simulink model "Dynamic_obstacle_avoidance"  (R2019a)
settings: Solver=VariableStepAuto  StartTime=0.0  StopTime=distance/V  MaxStep=1e-3  RelTol=1e-3  EnableMultiTasking=on
undefined symbols (not defined in the file): extended_map, Lw, obstacle, p, param, Ts, u0, WMV, WMVR, WOV, x0_dyn
libraries: simulink x2, mpclib x1
settings Model: Creator=The MathWorks, Inc.  LastModifiedBy=djtn
settings SolverCC: AlgebraicLoopSolver=LineSearch  MinimalZcImpactIntegration=on
settings DataIOCC: LimitDataPoints=on  SaveFormat=Array  SaveOutput=off  DSMLogging=off  SaveTime=off  ReturnWorkspaceOutputs=off
settings OptimizationCC: LifeSpan=inf
settings DebuggingCC: AlgebraicLoopMsg=none  UnderspecifiedInitializationDetection=Classic  MergeDetectMultiDrivingBlocksExec=none  SolverPrmCheckMsg=warning  AllowSymbolicDim=off  StateNameClashWarn=warning  SFUnexpectedBacktrackingDiag=warning  SFNoUnconditionalDefaultTransitionDiag=warning  SFExecutionAtInitializationDiag=none  UnderSpecifiedDimensionMsg=warning  ArithmeticOperatorsInVariantConditions=warning
settings HardwareCC: ProdBitPerPointer=32  ProdBitPerSizeT=32  ProdBitPerPtrDiffT=32  ProdLargestAtomicFloat=None  ProdIntDivRoundTo=Undefined  ProdEndianess=Unspecified  ProdWordSize=32  ProdHWDeviceType=32-bit Generic
settings ModelReferenceCC: PropagateSignalLabelsOutOfModel=off
settings SFSimCC: SimUseLocalCustomCode=off
settings RTWCC: RTWUseLocalCustomCode=off
settings CodeAppCC: StateflowObjectComments=on
settings GRTTargetCC: TargetLangStandard=C89/C90 (ANSI)
settings ConfigComp: CovMetricSettings=dw  CovSaveCumulativeToWorkspaceVar=on  CovSaveSingleToWorkspaceVar=on  CovExternalEMLEnable=off  CovSFcnEnable=off
settings SimscapeCC: SimscapeNormalizeSystem=off  SimscapeNominalValues="[{\"value\":\"10\",\"unit\":\"V\"},{\"value\":\"1\",\"unit\":\"A\"},{\"value\":\"10\",\"unit\":\"N*m\"},{\"value\":\"10\",\"unit\":\"bar\"},{\"value\":\"100\",\"unit\":\"kJ/kg\"},{\"value\":\"1\",\"unit\":\"kW\"},{\"value\":\"300\",\"unit\":\"K\"},{\"value\":\"100\",\"unit\":\"cm^3/s\"},{\"value\":\"1\",\"unit\":\"kN\"},{\"value\":\"1\",\"unit\":\"g/cm^3\"},{\"value\":\"1\",\"unit\":\"l\"},{\"value\":\"1\",\"unit\":\"cm^2\"},{\"value\":\"60\",\"unit\":\"Hz\"}]"
settings ConfigurationSet: Description=SimMechanics 2G
settings ExplorerConfigSet: InternalSimMechanicsExplorerSettings="<ExplorerConfiguration><canonicalview>default</canonicalview><AnimationSetting><BasePlaybackSpeed>1.0</BasePlaybackSpeed><PlaybackSpeedFactor>1.0</PlaybackSpeedFactor></AnimationSetting><TilePanel><TileInfo><Tiles Columns=\"1\" Count=\"1\" Rows=\"1\"><Column Left=\"2\" Weight=\"1\"/><Column Left=\"1552\"/><Row Top=\"2\" Weight=\"1\"/><Row Top=\"932\"/><Tile Height=\"1\" Width=\"1\" X=\"0\" Y=\"0\"/></Tiles></TileInfo><SceneInfo><SceneViewer><BGColor><R>0.60000002384185791</R><G>0.60000002384185791</G><B>0.60000002384185791</B></BGColor><Camera><Position><X>0.027865189060748197</X><Y>-2.5719092456962986</Y><Z>0.23157896538506753</Z></Position><Center><X>0.62659712312732463</X><Y>-0.46110119691712204</Y><Z>0.22087365386473376</Z></Center><Up><X>-0.0079438354874226333</X><Y>0.0073246425924307582</Y><Z>0.99994162084025784</Z></Up><Left>-0.24533778208815546</Left><Right>0.24533778208815546</Right><Bottom>-0.79734779727023208</Bottom><Top>0.79734779727023208</Top></Camera></SceneViewer></SceneInfo></TilePanel></ExplorerConfiguration>"

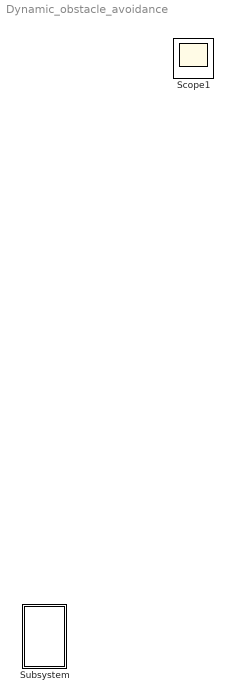
== system Dynamic_obstacle_avoidance ==
  Subsystem : Subsystem
  Scope1 : Scope

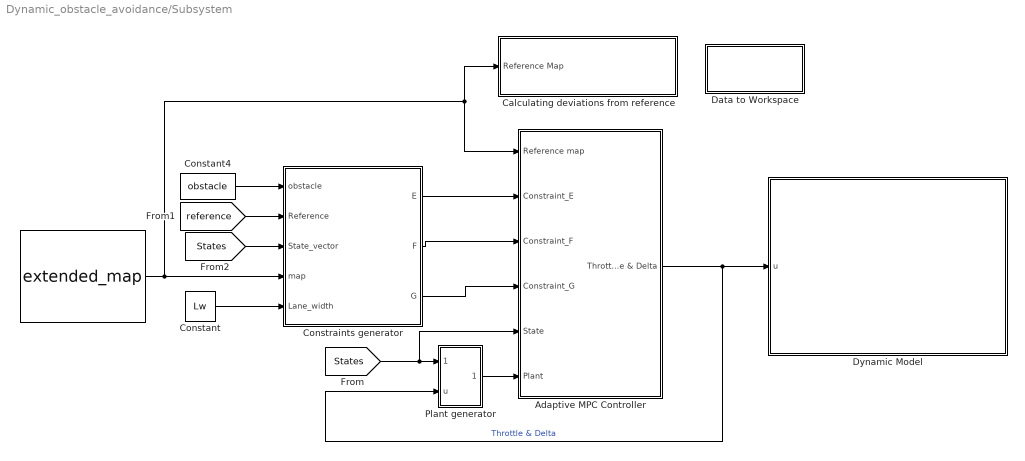
== system Dynamic_obstacle_avoidance/Subsystem ==
  "  " : Constant  Value=extended_map  SampleTime=Ts
      mask Display: image('creative_map_city.jpg')
  Adaptive MPC Controller : Subsystem
  Calculating deviations from reference : Subsystem
  Constant : Constant  Value=Lw
  Constant4 : Constant  Value=obstacle
  Constraints generator : Subsystem
  Data to Workspace : Subsystem
  Dynamic Model : Subsystem
      mask Display: image('hyundai_verna.jpg')
  Plant generator : Subsystem
  wires:
  Plant generator/1(Out1) -> Adaptive MPC Controller/6(Plant)
  Constraints generator/3(G) -> Adaptive MPC Controller/4(Constraint_G)
  "  "/1 -> Adaptive MPC Controller/1(Reference map), Calculating deviations from reference/1(Reference Map), Constraints generator/4(map)
  Adaptive MPC Controller/1(Throttle & Delta) -> Dynamic Model/1(u), Plant generator/2(u)  "Throttle & Delta"
  Constraints generator/1(E) -> Adaptive MPC Controller/2(Constraint_E)
  Constraints generator/2(F) -> Adaptive MPC Controller/3(Constraint_F)
  [States] -> Adaptive MPC Controller/5(State), Plant generator/1(State)
  Constant4/1 -> Constraints generator/1(obstacle)
  [reference] -> Constraints generator/2(Reference)
  Constant/1 -> Constraints generator/5(Lane_width)
  [States] -> Constraints generator/3(State_vector)

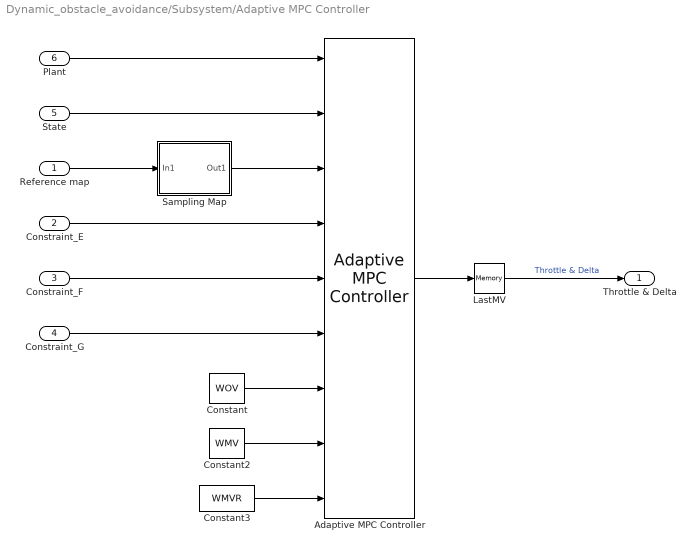
== system Dynamic_obstacle_avoidance/Subsystem/Adaptive MPC Controller ==
  Reference map : Inport
  Constraint_E : Inport  Port=2
  Constraint_F : Inport  Port=3
  Constraint_G : Inport  Port=4
  State : Inport  Port=5
  Plant : Inport  Port=6
  Adaptive MPC Controller : mpclib/Adaptive MPC Controller  SCDEnableBlockLinearizationSpecification=on  mpcobj=mpcobj  x0=egoStates  enable_value=0  updateMPCinCallerWorkspace=on  md_inport=off  mv_inport=off  uref_inport=off  return_cost=off  return_mvseq=off  return_qpstatus=off  return_xseq=off  return_state=off  return_ovseq=off  state_inport=off  isltv_plant=off  umin_inport=off  umax_inport=off  ymin_inport=off  ymax_inport=off  cc_inport=on  ywt_inport=on  uwt_inport=on  duwt_inport=on  rhoeps_inport=off  pm_inport=off  MaximumP=10  HorizonChoice=FixedHorizon  BlockDataType=double  SampleTimeInherited=on  switch_inport=off
  Constant : Constant  Value=WOV
  Constant2 : Constant  Value=WMV
  Constant3 : Constant  Value=WMVR
  LastMV : Memory  InitialCondition=u0
  Sampling Map : Subsystem
  Throttle & Delta : Outport  VectorParamsAs1DForOutWhenUnconnected=on
  wires:
  Constraint_E/1 -> Adaptive MPC Controller/4
  Constraint_G/1 -> Adaptive MPC Controller/6
  Constant3/1 -> Adaptive MPC Controller/9
  Constant2/1 -> Adaptive MPC Controller/8
  Constraint_F/1 -> Adaptive MPC Controller/5
  Constant/1 -> Adaptive MPC Controller/7
  State/1 -> Adaptive MPC Controller/2
  Adaptive MPC Controller/1 -> LastMV/1
  LastMV/1 -> Throttle & Delta/1  "Throttle & Delta"
  Plant/1 -> Adaptive MPC Controller/1
  Reference map/1 -> Sampling Map/1(In1)
  Sampling Map/1(Out1) -> Adaptive MPC Controller/3

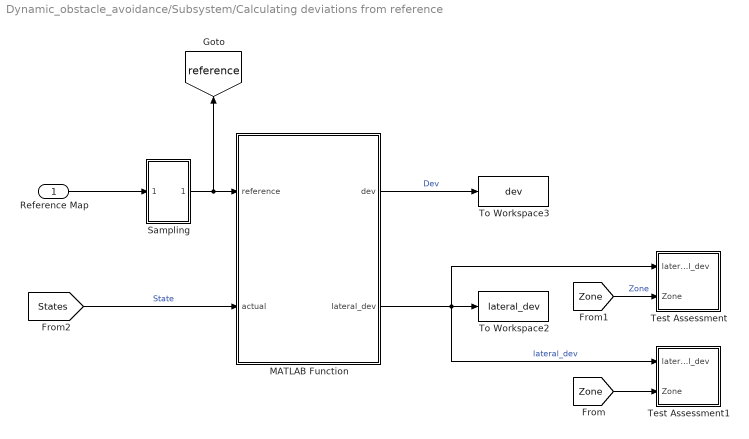
== system Dynamic_obstacle_avoidance/Subsystem/Calculating deviations from reference ==
  Reference Map : Inport
  MATLAB Function : MATLAB Function  TreatAsAtomicUnit=on
  Sampling : Subsystem
  Test Assessment : Test Sequence  TreatAsAtomicUnit=on
  Test Assessment1 : Test Sequence  TreatAsAtomicUnit=on
  To Workspace2 : ToWorkspace  VariableName=lateral_dev  SampleTime=Ts
  To Workspace3 : ToWorkspace  VariableName=dev  SampleTime=-1
  tag scope: reference=global
  wires:
  [Zone] -> Test Assessment1/2(Zone)
  [Zone] -> Test Assessment/2(Zone)  "Zone"
  MATLAB Function/2(lateral_dev) -> To Workspace2/1, Test Assessment/1(lateral_dev), Test Assessment1/1(lateral_dev)  "lateral_dev"
  MATLAB Function/1(dev) -> To Workspace3/1  "Dev"
  [States] -> MATLAB Function/2(actual)  "State"
  Reference Map/1 -> Sampling/1(In1)
  Sampling/1(Out1) -> MATLAB Function/1(reference), [reference]

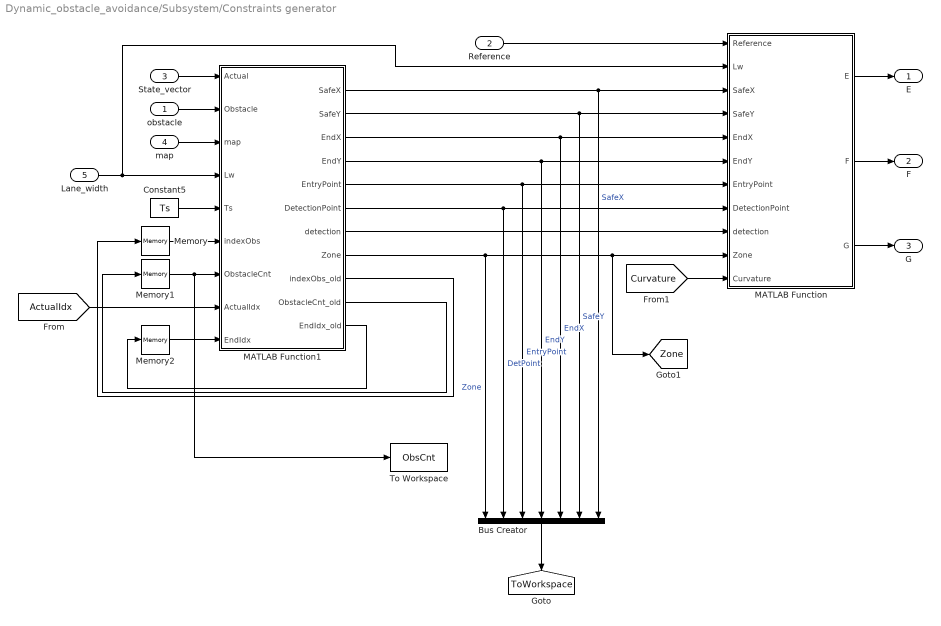
== system Dynamic_obstacle_avoidance/Subsystem/Constraints generator ==
  obstacle : Inport
  Reference : Inport  Port=2
  State_vector : Inport  Port=3
  map : Inport  Port=4
  Lane_width : Inport  Port=5
  Bus Creator : BusCreator  Inputs=7
  Constant5 : Constant  Value=Ts
  MATLAB Function : MATLAB Function  TreatAsAtomicUnit=on
  MATLAB Function1 : MATLAB Function  TreatAsAtomicUnit=on
  Memory : Memory
  Memory1 : Memory
  Memory2 : Memory
  To Workspace : ToWorkspace  VariableName=ObsCnt  SampleTime=Ts
  E : Outport  VectorParamsAs1DForOutWhenUnconnected=on
  F : Outport  Port=2  VectorParamsAs1DForOutWhenUnconnected=on
  G : Outport  Port=3  VectorParamsAs1DForOutWhenUnconnected=on
  tag scope: ToWorkspace=global, Zone=global
  wires:
  obstacle/1 -> MATLAB Function1/2(Obstacle)
  State_vector/1 -> MATLAB Function1/1(Actual)
  map/1 -> MATLAB Function1/3(map)
  Constant5/1 -> MATLAB Function1/5(Ts)
  Lane_width/1 -> MATLAB Function1/4(Lw), MATLAB Function/2(Lw)
  Memory/1 -> MATLAB Function1/6(indexObs)
  MATLAB Function1/9(indexObs_old) -> Memory/1
  MATLAB Function1/1(SafeX) -> Bus Creator/7, MATLAB Function/3(SafeX)  "SafeX"
  MATLAB Function1/2(SafeY) -> Bus Creator/6, MATLAB Function/4(SafeY)  "SafeY"
  MATLAB Function1/3(EndX) -> Bus Creator/5, MATLAB Function/5(EndX)  "EndX"
  MATLAB Function1/4(EndY) -> Bus Creator/4, MATLAB Function/6(EndY)  "EndY"
  MATLAB Function1/5(EntryPoint) -> Bus Creator/3, MATLAB Function/7(EntryPoint)  "EntryPoint"
  MATLAB Function1/6(DetectionPoint) -> Bus Creator/2, MATLAB Function/8(DetectionPoint)  "DetPoint"
  MATLAB Function1/7(detection) -> MATLAB Function/9(detection)
  MATLAB Function1/8(Zone) -> Bus Creator/1, MATLAB Function/10(Zone), [Zone]  "Zone"
  Reference/1 -> MATLAB Function/1(Reference)
  MATLAB Function/1(E) -> E/1
  MATLAB Function/2(F) -> F/1
  MATLAB Function/3(G) -> G/1
  Memory1/1 -> To Workspace/1, MATLAB Function1/7(ObstacleCnt)
  MATLAB Function1/10(ObstacleCnt_old) -> Memory1/1
  [ActualIdx] -> MATLAB Function1/8(ActualIdx)
  Memory2/1 -> MATLAB Function1/9(EndIdx)
  MATLAB Function1/11(EndIdx_old) -> Memory2/1
  Bus Creator/1 -> [ToWorkspace]
  [Curvature] -> MATLAB Function/11(Curvature)

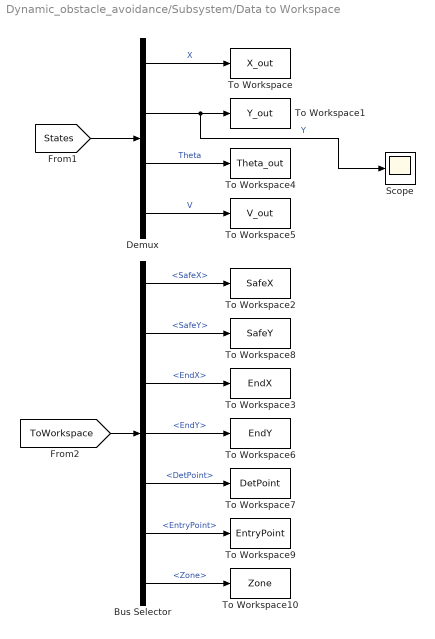
== system Dynamic_obstacle_avoidance/Subsystem/Data to Workspace ==
  Bus Selector : BusSelector  OutputSignals=SafeX,SafeY,EndX,EndY,DetPoint,EntryPoint,Zone
  Demux : Demux
  Scope : Scope
  To Workspace : ToWorkspace  VariableName=X_out  SampleTime=-1
  To Workspace1 : ToWorkspace  VariableName=Y_out  SampleTime=-1
  To Workspace10 : ToWorkspace  VariableName=Zone  SampleTime=-1
  To Workspace2 : ToWorkspace  VariableName=SafeX  SampleTime=-1
  To Workspace3 : ToWorkspace  VariableName=EndX  SampleTime=-1
  To Workspace4 : ToWorkspace  VariableName=Theta_out  SampleTime=-1
  To Workspace5 : ToWorkspace  VariableName=V_out  SampleTime=-1
  To Workspace6 : ToWorkspace  VariableName=EndY  SampleTime=-1
  To Workspace7 : ToWorkspace  VariableName=DetPoint  SampleTime=-1
  To Workspace8 : ToWorkspace  VariableName=SafeY  SampleTime=-1
  To Workspace9 : ToWorkspace  VariableName=EntryPoint  SampleTime=-1
  wires:
  Demux/3 -> To Workspace4/1  "Theta"
  Demux/2 -> Scope/1, To Workspace1/1  "Y"
  Demux/4 -> To Workspace5/1  "V"
  [States] -> Demux/1
  Demux/1 -> To Workspace/1  "X"
  [ToWorkspace] -> Bus Selector/1
  Bus Selector/1 -> To Workspace2/1  "<SafeX>"
  Bus Selector/2 -> To Workspace8/1  "<SafeY>"
  Bus Selector/3 -> To Workspace3/1  "<EndX>"
  Bus Selector/4 -> To Workspace6/1  "<EndY>"
  Bus Selector/5 -> To Workspace7/1  "<DetPoint>"
  Bus Selector/6 -> To Workspace9/1  "<EntryPoint>"
  Bus Selector/7 -> To Workspace10/1  "<Zone>"

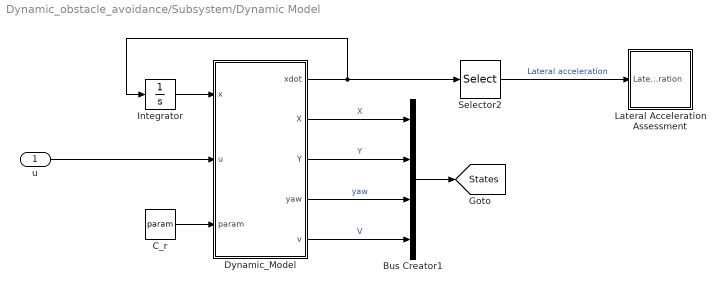
== system Dynamic_obstacle_avoidance/Subsystem/Dynamic Model ==
  u : Inport
  Bus Creator1 : BusCreator  Inputs=4
  C_r : Constant  Value=param  SampleTime=Ts
  Dynamic_Model : MATLAB Function  TreatAsAtomicUnit=on
  Integrator : Integrator  InitialCondition=x0_dyn
  Lateral Acceleration Assessment : Test Sequence  TreatAsAtomicUnit=on
  Selector2 : Selector  InputPortWidth=6  IndexOptions=Index vector (dialog)  Indices=[5]  OutputSizes=1
  tag scope: States=global
  wires:
  Dynamic_Model/3(Y) -> Bus Creator1/2  "Y"
  Bus Creator1/1 -> [States]
  Selector2/1 -> Lateral Acceleration Assessment/1(Lateral_acceleration)  "Lateral acceleration"
  Dynamic_Model/1(xdot) -> Integrator/1, Selector2/1
  Dynamic_Model/4(yaw) -> Bus Creator1/3  "yaw"
  Dynamic_Model/2(X) -> Bus Creator1/1  "X"
  Dynamic_Model/5(v) -> Bus Creator1/4  "V"
  Integrator/1 -> Dynamic_Model/1(x)
  C_r/1 -> Dynamic_Model/3(param)
  u/1 -> Dynamic_Model/2(u)

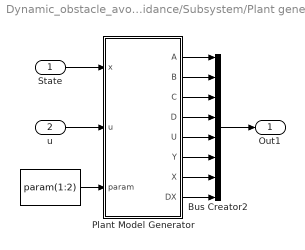
== system Dynamic_obstacle_avoidance/Subsystem/Plant generator ==
  State : Inport
  u : Inport  Port=2
  " " : Constant  Value=param(1:2)  SampleTime=Ts
  Bus Creator2 : BusCreator  Inputs=8
  Plant Model Generator : MATLAB Function  TreatAsAtomicUnit=on
  Out1 : Outport  VectorParamsAs1DForOutWhenUnconnected=on
  wires:
  " "/1 -> Plant Model Generator/3(param)
  Plant Model Generator/6(Y) -> Bus Creator2/6
  Plant Model Generator/3(C) -> Bus Creator2/3
  Plant Model Generator/2(B) -> Bus Creator2/2
  Plant Model Generator/7(X) -> Bus Creator2/7
  u/1 -> Plant Model Generator/2(u)
  Plant Model Generator/5(U) -> Bus Creator2/5
  Plant Model Generator/4(D) -> Bus Creator2/4
  Plant Model Generator/1(A) -> Bus Creator2/1
  Plant Model Generator/8(DX) -> Bus Creator2/8
  Bus Creator2/1 -> Out1/1
  State/1 -> Plant Model Generator/1(x)

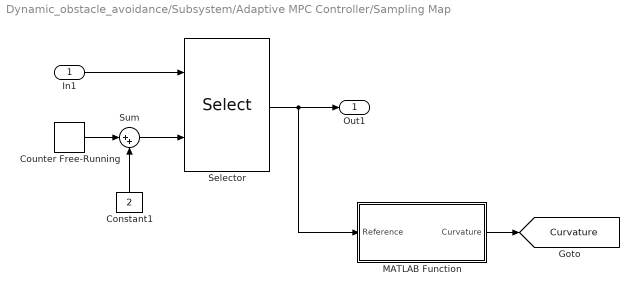
== system Dynamic_obstacle_avoidance/Subsystem/Adaptive MPC Controller/Sampling Map ==
  In1 : Inport
  Constant1 : Constant  Value=2
  Counter Free-Running : simulink/Sources/Counter Free-Running  NumBits=32  tsamp=Ts
  MATLAB Function : MATLAB Function  TreatAsAtomicUnit=on
  Selector : Selector  NumberOfDimensions=2  InputPortWidth=3  IndexOptions=Starting index (port),Select all  Indices=[1 3],1  OutputSizes=p,1
  Sum : Sum  Inputs=|++
  Out1 : Outport  VectorParamsAs1DForOutWhenUnconnected=on
  tag scope: Curvature=global
  wires:
  Selector/1 -> MATLAB Function/1(Reference), Out1/1
  In1/1 -> Selector/1
  Counter Free-Running/1 -> Sum/1
  Sum/1 -> Selector/2
  Constant1/1 -> Sum/2
  MATLAB Function/1(Curvature) -> [Curvature]

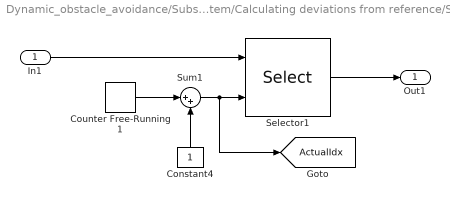
== system Dynamic_obstacle_avoidance/Subsystem/Calculating deviations from reference/Sampling ==
  In1 : Inport
  Constant4 : Constant
  Counter Free-Running1 : simulink/Sources/Counter Free-Running  NumBits=32  tsamp=Ts
  Selector1 : Selector  NumberOfDimensions=2  InputPortWidth=3  IndexOptions=Starting index (port),Select all  Indices=[1 3],1  OutputSizes=1,1
  Sum1 : Sum  Inputs=|++
  Out1 : Outport  VectorParamsAs1DForOutWhenUnconnected=on
  tag scope: ActualIdx=global
  wires:
  Counter Free-Running1/1 -> Sum1/1
  Constant4/1 -> Sum1/2
  Sum1/1 -> [ActualIdx], Selector1/2
  Selector1/1 -> Out1/1
  In1/1 -> Selector1/1

== matlab function Dynamic_obstacle_avoidance/Subsystem/Adaptive MPC Controller/Sampling Map/MATLAB Function ==
  data: Reference input; Curvature output
function Curvature = fcn(Reference)

Curvature = curvatureEstimator(Reference);

== matlab function Dynamic_obstacle_avoidance/Subsystem/Calculating deviations from reference/MATLAB Function ==
  settings: updateMethod=DISCRETE  sampleTime=Ts
  data: reference input; dev output; actual input; lateral_dev output
function [dev,lateral_dev] = fcn(reference, actual)

[dev, lateral_dev] = deviation(reference,actual);

== stateflow chart Dynamic_obstacle_avoidance/Subsystem/Calculating deviations from reference/Test Assessment ==
  settings: stateMachineType=SIMPLIFIED_MACHINE
  state Left_Lane_assessment
    if Zone == 3
    verify(lateral_dev >= 2 && lateral_dev <= 6);
    elseif Zone == 2 || Zone == 4
    verify(lateral_dev < 6)
    end
  (default) -> Left_Lane_assessment
  data: lateral_dev input; Zone input

== stateflow chart Dynamic_obstacle_avoidance/Subsystem/Calculating deviations from reference/Test Assessment1 ==
  settings: stateMachineType=SIMPLIFIED_MACHINE
  state Safe_Overtake_Assessment
    if Zone == 3
    verify(duration(lateral_dev > 5 && lateral_dev < 3,sec)<1);
    end
  (default) -> Safe_Overtake_Assessment
  data: lateral_dev input; Zone input

== matlab function Dynamic_obstacle_avoidance/Subsystem/Constraints generator/MATLAB Function ==
  settings: updateMethod=DISCRETE  sampleTime=Ts
  data: Reference input; E output size=[2 2]; Lw input; SafeX input; SafeY input; EndX input; EndY input; EntryPoint input; DetectionPoint input; detection input; F output size=[2 4]; G output size=[2 1]; Zone input; Curvature input
function [E, F, G] = fcn(Reference,Lw,SafeX,SafeY,EndX,EndY,EntryPoint,DetectionPoint,detection,Zone,Curvature)

[E, F, G] = LaneKeepConstraint(Reference,Lw,detection,SafeX,SafeY,EndX,EndY,EntryPoint,Zone,DetectionPoint,Curvature);

== matlab function Dynamic_obstacle_avoidance/Subsystem/Constraints generator/MATLAB Function1 ==
  settings: updateMethod=DISCRETE  sampleTime=Ts
  data: Actual input; SafeX output; Obstacle input; SafeY output; EndX output; EndY output; EntryPoint output; DetectionPoint output; detection output; map input; Lw input; Ts input; Zone output; indexObs input; indexObs_old output; ObstacleCnt_old output; ObstacleCnt input; ActualIdx input; EndIdx input; EndIdx_old output
function [SafeX,SafeY,EndX,EndY,EntryPoint,DetectionPoint,detection,Zone,indexObs_old,ObstacleCnt_old,EndIdx_old] = fcn(Actual,Obstacle,map,Lw,Ts,indexObs,ObstacleCnt,ActualIdx,EndIdx)

[SafeX,SafeY,EndX,EndY,EntryPoint,detection,Zone,indexObs_old,DetectionPoint,ObstacleCnt_old,EndIdx_old] = detectionFun(Actual,Obstacle,map,Lw,Ts,indexObs,ObstacleCnt,ActualIdx,EndIdx);

== matlab function Dynamic_obstacle_avoidance/Subsystem/Dynamic Model/Dynamic_Model ==
  data: x input; u input; xdot output; param input; X output; Y output; yaw output; v output
function [xdot,X, Y, yaw, v] = fcn(x,u,param)

[xdot,X, Y, yaw, v] = VehicleModelCT_DYN(x,u,param);

== stateflow chart Dynamic_obstacle_avoidance/Subsystem/Dynamic Model/Lateral Acceleration Assessment ==
  settings: stateMachineType=SIMPLIFIED_MACHINE
  state Global_Assessment
    % Check if the lateral acceleration of the vehicle is below 2m/s^2  except for half a second period
    verify(duration(Lateral_acceleration>=2,sec)<=0.5)
  (default) -> Global_Assessment
  data: Lateral_acceleration input

== matlab function Dynamic_obstacle_avoidance/Subsystem/Plant generator/Plant Model Generator ==
  settings: updateMethod=DISCRETE  sampleTime=Ts
  data: x input; u input; A output; B output; C output; D output; U output size=[2,1]; Y output size=[4,1]; X output size=[4,1]; DX output size=[4,1]; Ts parameter; param input
function [A,B,C,D,U,Y,X,DX] = fcn(x,u,Ts,param)
[A,B,C,D,U,Y,X,DX] = obstacleVehicleModelDT(Ts,x,u,param);
